simulink model "lab3ol"  (Simulink 7.3)
settings: Solver=ode45  StartTime=0.0  StopTime=20.0  RelTol=1e-3
settings Model: Creator=Mark  LastModifiedBy=linsong
settings OptimizationCC: InlineInvariantSignals=on  InitFltsAndDblsToZero=on
settings DebuggingCC: SaveWithParameterizedLinksMsg=none  SignalResolutionControl=TryResolveAllWithWarning  MultiTaskDSMMsg=warning  MultiTaskCondExecSysMsg=none  StrictBusMsg=None
settings RTWCC: IncludeERTFirstTime=on
settings GRTTargetCC: TargetFcnLib=ansi_tfl_tmw.mat

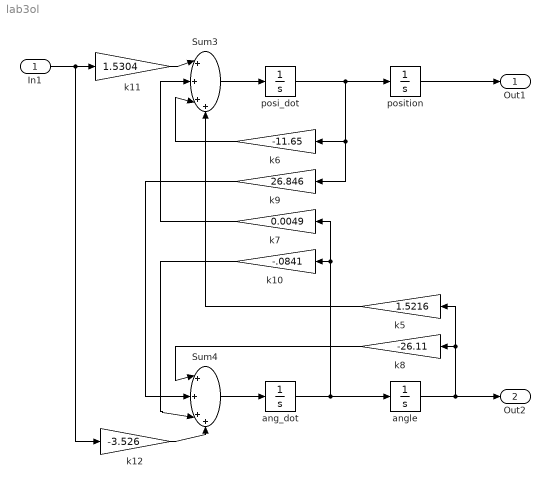
== system lab3ol ==
  In1 : Inport  OutDataType=fixdt(1, 16)  OutScaling=2^0
  Sum3 : Sum  Inputs=|++++  OutDataType=sfix(16)  OutScaling=2^0
  Sum4 : Sum  Inputs=|++++  OutDataType=sfix(16)  OutScaling=2^0
  ang_dot : Integrator
  angle : Integrator
  k10 : Gain  Gain=-.0841  ParameterDataType=sfix(16)  ParameterScaling=2^0  OutDataType=sfix(16)  OutScaling=2^0
  k11 : Gain  Gain=1.5304  ParameterDataType=sfix(16)  ParameterScaling=2^0  OutDataType=sfix(16)  OutScaling=2^0
  k12 : Gain  Gain=-3.526  ParameterDataType=sfix(16)  ParameterScaling=2^0  OutDataType=sfix(16)  OutScaling=2^0
  k5 : Gain  Gain=1.5216  ParameterDataType=sfix(16)  ParameterScaling=2^0  OutDataType=sfix(16)  OutScaling=2^0
  k6 : Gain  Gain=-11.65  ParameterDataType=sfix(16)  ParameterScaling=2^0  OutDataType=sfix(16)  OutScaling=2^0
  k7 : Gain  Gain=0.0049  ParameterDataType=sfix(16)  ParameterScaling=2^0  OutDataType=sfix(16)  OutScaling=2^0
  k8 : Gain  Gain=-26.11  ParameterDataType=sfix(16)  ParameterScaling=2^0  OutDataType=sfix(16)  OutScaling=2^0
  k9 : Gain  Gain=26.846  ParameterDataType=sfix(16)  ParameterScaling=2^0  OutDataType=sfix(16)  OutScaling=2^0
  posi_dot : Integrator
  position : Integrator
  Out1 : Outport  OutDataType=sfix(16)  OutScaling=2^0
  Out2 : Outport  Port=2  OutDataType=sfix(16)  OutScaling=2^0
  wires:
  position/1 -> Out1/1
  Sum3/1 -> posi_dot/1
  Sum4/1 -> ang_dot/1
  angle/1 -> k8/1, k5/1, Out2/1
  ang_dot/1 -> angle/1, k10/1, k7/1
  k5/1 -> Sum3/4
  k8/1 -> Sum4/1
  k6/1 -> Sum3/3
  k9/1 -> Sum4/2
  k7/1 -> Sum3/2
  k10/1 -> Sum4/3
  k11/1 -> Sum3/1
  k12/1 -> Sum4/4
  posi_dot/1 -> position/1, k6/1, k9/1
  In1/1 -> k11/1, k12/1
